simulink model "Blink_LED_Logging"  (R2024b)
settings: Solver=FixedStepAuto  StartTime=0.0  StopTime=inf  RelTol=1e-3  EnableMultiTasking=on
libraries: stm32f4xxblockslib x3, simulink x2
settings Model: STM32="{\"DigitalPortWrite\":{\"ID\":\"motor_control:4\"},\"DigitalPortRead\":{\"ID\":\"motor_control:3\"},\"HardwareInterrupt\":{\"ID\":\"motor_control:31\"}}"  SimulationMode=external  ExtModeEnableFloating=off  Creator=sakee  LastModifiedBy=sakee
settings SolverCC: AutoInsertRateTranBlk=on
settings OptimizationCC: EnhancedBackFolding=on  PassReuseOutputArgsAs=Individual arguments  ZeroExternalMemoryAtStartup=off  ZeroInternalMemoryAtStartup=off  MaxStackSize=512  OptimizeBlockOrder=speed  DifferentSizesBufferReuse=on  OptimizationCustomize=off  EfficientTunableParamExpr=on
settings DebuggingCC: ParameterTunabilityLossMsg=error
settings HardwareCC: ProdBitPerPointer=32  ProdBitPerSizeT=32  ProdBitPerPtrDiffT=32  ProdLargestAtomicInteger=Long  ProdLargestAtomicFloat=Double  ProdWordSize=32  ProdLongLongMode=on  ProdHWDeviceType=ARM Compatible->ARM Cortex-M
settings SFSimCC: MATLABDynamicMemAlloc=off
settings RTWCC: Description=Embedded Coder  SystemTargetFile=ert.tlc  HardwareBoard=STM32F4xx Based  TemplateMakefile=ert_default_tmf  Toolchain=GNU Tools for ARM Embedded Processors
settings CodeAppCC: ForceParamTrailComments=on  IgnoreCustomStorageClasses=off  OperatorAnnotations=on  SimulinkDataObjDesc=on  SFDataObjDesc=on  InsertBlockDesc=on
settings ERTTargetCC: TargetLangStandard=C99 (ISO)  CodeReplacementLibrary=ARM Cortex-M  ExtModeTransport=3  ExtModeStaticAlloc=on  ExtModeStaticAllocSize=2048  ExtModeMexFile=ext_xcp  ExtModeIntrfLevel=Level2 - Open  InlinedParameterPlacement=Hierarchical

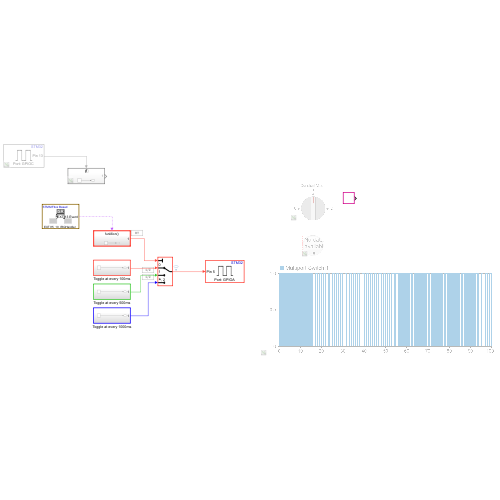
[thumbnail: Simulink's stored preview of the top-level diagram]
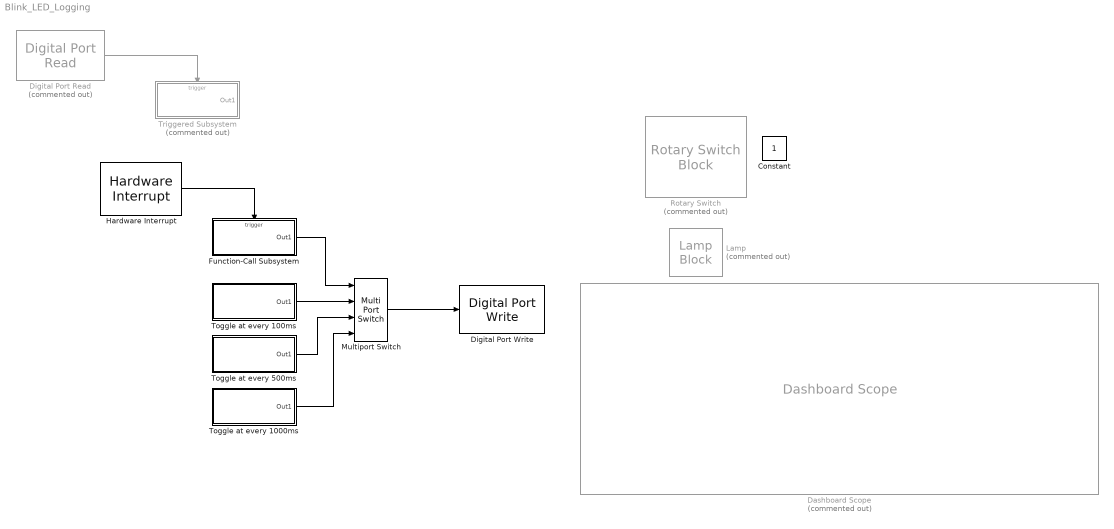
== system Blink_LED_Logging ==
  Constant : Constant
  Dashboard Scope : DashboardScope  Commented=on  Ymin=0  Ymax=1
  Digital Port Read : stm32f4xxblockslib/Digital Port Read  Commented=on  PortName=GPIOC  PinNumber=13  ReadOperation=on  IOAsArray=off  SampleTime=-1  EnableSimPort=off  hoistedMaskSrc=ECSoC/ECSimCodegen/Digital Port Read
  Digital Port Write : stm32f4xxblockslib/Digital Port Write  PortName=GPIOA  PinNumber=5  ReadOperation=off  IOAsArray=off  EnableSimPort=off  hoistedMaskSrc=ECSoC/ECSimCodegen/Digital Port Write
  Function-Call Subsystem : Subsystem  TreatAsAtomicUnit=on
  Hardware Interrupt : stm32f4xxblockslib/Hardware Interrupt  ISRGroup=External interrupts (EXTI)  ISRName=EXTI15_10_IRQHandler  ISRNumber=55  EventsList={ 'off', 'EXTI15 Event', '1'; 'off', 'EXTI14 Event', '2'; 'on', 'EXTI13 Event', '3'; 'off', 'EXTI12 Event', '4'; 'off', 'EXTI11 Event', '5'; 'off', 'EXTI10 Event', '6'; 'off', 'Custom event', '7' }  SelectedEvents={'EXTI13 Event'}  TaskPriority=30  DisablePreemption=off  ClearInterruptFlagsAtEndOfEvent=off  InterruptDefinitionFile=$(TARGET_ROOT)/registry/interrupts/STM32F4xxBased_interrupts.xml  HardwareBoard=STM32F4xx Based  EnableSimPort=off
  Lamp : LampBlock  Commented=on  LabelPosition=Hide
  Multiport Switch : MultiPortSwitch  DataPortOrder=Zero-based contiguous  zeroidx=on  SaturateOnIntegerOverflow=off  InputSameDT=off
  Rotary Switch : RotarySwitchBlock  Commented=on
      settings: Values={{'0', '1', '2'}, [0 1 2]}
  Toggle at every 1000ms : Subsystem
  Toggle at every 100ms : Subsystem
  Toggle at every 500ms : Subsystem
  Triggered Subsystem : Subsystem  Commented=on  TreatAsAtomicUnit=on
  wires:
  Toggle at every 500ms/1(Out1) -> Multiport Switch/3
  Toggle at every 1000ms/1(Out1) -> Multiport Switch/4
  Toggle at every 100ms/1(Out1) -> Multiport Switch/2
  Multiport Switch/1 -> Digital Port Write/1
  Digital Port Read/1 -> Triggered Subsystem/Trigger
  Function-Call Subsystem/1(Out1) -> Multiport Switch/1
  Hardware Interrupt/1 -> Function-Call Subsystem/Trigger

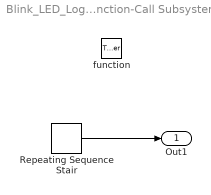
== system Blink_LED_Logging/Function-Call Subsystem ==
  function : TriggerPort  TriggerType=function-call  VariantControl=(inherit)
  Repeating Sequence Stair : simulink/Sources/Repeating Sequence Stair  OutValues=[1 2 0]  tsamp=-1  OutMin=[]  OutMax=[]  OutDataTypeStr=double  OutputDataTypeScalingMode=double  OutDataType=fixdt(0,8)  ConRadixGroup=Best Precision: Vector-wise  OutScaling=2^-12
  Out1 : Outport
  wires:
  Repeating Sequence Stair/1 -> Out1/1

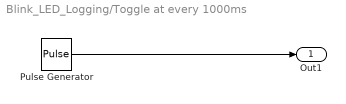
== system Blink_LED_Logging/Toggle at every 1000ms ==
  Pulse Generator : DiscretePulseGenerator
  Out1 : Outport
  wires:
  Pulse Generator/1 -> Out1/1

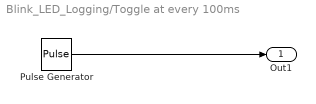
== system Blink_LED_Logging/Toggle at every 100ms ==
  Pulse Generator : DiscretePulseGenerator  SampleTime=0.1
  Out1 : Outport
  wires:
  Pulse Generator/1 -> Out1/1

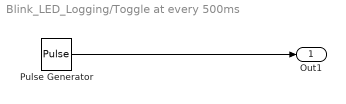
== system Blink_LED_Logging/Toggle at every 500ms ==
  Pulse Generator : DiscretePulseGenerator  SampleTime=0.5
  Out1 : Outport
  wires:
  Pulse Generator/1 -> Out1/1

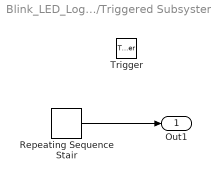
== system Blink_LED_Logging/Triggered Subsystem ==
  Trigger : TriggerPort  VariantControl=(inherit)
  Repeating Sequence Stair : simulink/Sources/Repeating Sequence Stair  OutValues=[1 2 0]  tsamp=-1  OutMin=[]  OutMax=[]  OutDataTypeStr=double  OutputDataTypeScalingMode=double  OutDataType=fixdt(0,8)  ConRadixGroup=Best Precision: Vector-wise  OutScaling=2^-12
  Out1 : Outport
  wires:
  Repeating Sequence Stair/1 -> Out1/1
